simulink model "Image_Processing"  (Simulink 7.5)
settings: Solver=ode45  StartTime=0.0  StopTime=10.0  RelTol=1e-3
undefined symbols (not defined in the file or in its folder): gray
libraries: dspsrcs4 x1, vipsnks x1
settings Model: Creator=roczit00  LastModifiedBy=Dio
settings DebuggingCC: StrictBusMsg=Warning

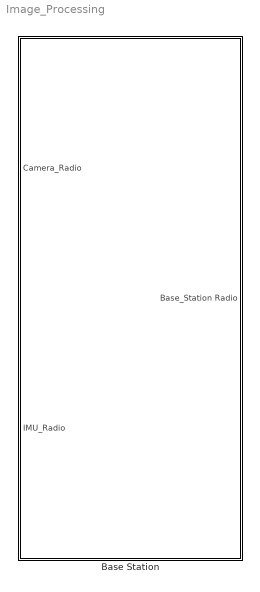
== system Image_Processing ==
  Base Station : Subsystem

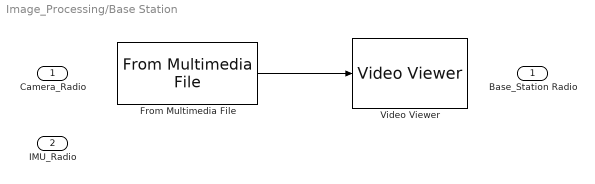
== system Image_Processing/Base Station ==
  Camera_Radio : Inport  OutDataType=fixdt(1, 16)  OutScaling=2^0
  IMU_Radio : Inport  Port=2  OutDataType=fixdt(1, 16)  OutScaling=2^0
  From Multimedia File : dspsrcs4/From Multimedia File  DialogController=dspDDGCreate  DialogControllerArgs=DataTag0  inputFilename=D:\_HSE\_ARBEIT\eclipse-cpp-galileo-SR1-win32\Workspace2\MASTER_THESIS_PRJ\scratch\Ground_Videos\grey_amorphic_flow_tiles_variable_light.avi  loop=on  numPlays=inf  outputStreams=Video only  videoDataType=single  audioDataType=int16  inheritSampleTime=on  userDefinedSampleTime=1/30  noAudioOutput=off  isIntensityVideo=off  fourcc=RGB  colorVideoFormat=One multidimensional signal  outputEOF=off  dataOrg=Column-major  audioFrameSize=1024  computeAudioFrameSize=off
  Video Viewer : vipsnks/Video Viewer  DialogControllerArgs=DataTag2  inputType=Obsolete7b  imagePorts=One multidimensional signal  useColorMap=off  colormapValue=gray(256)  specRange=off  minInputVal=0  maxInputVal=255  FigPos=[755 449 410 300]  AxisZoom=on  trueSizedOnce=off  OpenAtMdlStart=on
  Base_Station Radio : Outport  OutDataType=fixdt(1, 16)  OutScaling=2^0
  wires:
  From Multimedia File/1 -> Video Viewer/1
